simulink model "termicD1"  (Simulink 7.2)
settings: Solver=ode45  StartTime=0.0  StopTime=7000.0  RelTol=1e-3
undefined symbols (not defined in the file): T
libraries: simulink x2
settings Model: Creator=dpara  LastModifiedBy=dpara

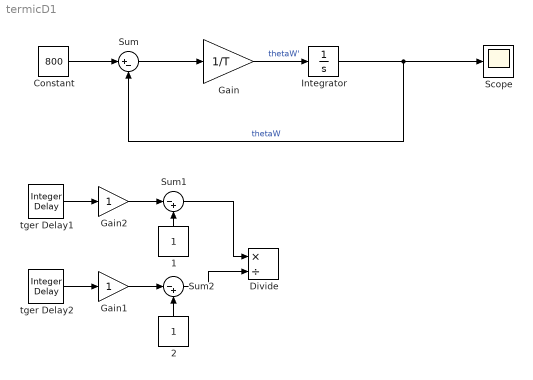
== system termicD1 ==
  1 : Constant  Orientation=up  OutDataType=sfix(16)  OutScaling=2^0
  2 : Constant  Orientation=up  OutDataType=sfix(16)  OutScaling=2^0
  Constant : Constant  Value=800  OutDataType=sfix(16)  OutScaling=2^0
  Divide : Product  Inputs=*/  OutDataType=sfix(16)  OutScaling=2^-10
  Gain : Gain  Gain=1/T  ParameterDataType=sfix(16)  ParameterScaling=2^0  OutDataType=sfix(16)  OutScaling=2^0
  Gain1 : Gain  ParameterDataType=sfix(16)  ParameterScaling=2^0  OutDataType=sfix(16)  OutScaling=2^0
  Gain2 : Gain  ParameterDataType=sfix(16)  ParameterScaling=2^0  OutDataType=sfix(16)  OutScaling=2^0
  Integrator : Integrator  InitialCondition=20
  Scope : Scope
  Sum : Sum  Inputs=|+-  OutDataType=sfix(16)  OutScaling=2^0
  Sum1 : Sum  Inputs=|-+  OutDataType=sfix(16)  OutScaling=2^0
  Sum2 : Sum  Inputs=|-+  OutDataType=sfix(16)  OutScaling=2^0
  tger Delay1 : simulink/Discrete/Integer Delay  vinit=0.0  samptime=-1  NumDelays=1
  tger Delay2 : simulink/Discrete/Integer Delay  vinit=0.0  samptime=-1  NumDelays=1
  wires:
  Sum/1 -> Gain/1
  Gain2/1 -> Sum1/1
  Sum1/1 -> Divide/1
  tger Delay1/1 -> Gain2/1
  1/1 -> Sum1/2
  Gain1/1 -> Sum2/1
  tger Delay2/1 -> Gain1/1
  2/1 -> Sum2/2
  Sum2/1 -> Divide/2
  Constant/1 -> Sum/1
  Gain/1 -> Integrator/1  "thetaW'"
  Integrator/1 -> Scope/1, Sum/2  "thetaW"
